simulink model "TypesOfSolverr"  (R2013a)
settings: Solver=FixedStepDiscrete  StartTime=0  StopTime=20  FixedStep=1  MaxStep=1  RelTol=1e-3
settings Model: Creator=ajdin  LastModifiedBy=ajdin
settings DataIOCC: LoadExternalInput=on

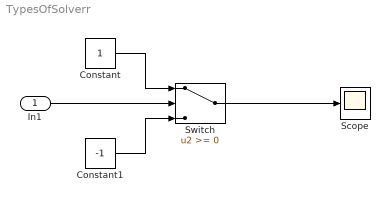
== system TypesOfSolverr ==
  In1 : Inport
  Constant : Constant
  Constant1 : Constant  Value=-1
  Scope : Scope
      settings: YMin=-3  YMax=3
  Switch : Switch
  wires:
  Switch/1 -> Scope/1
  In1/1 -> Switch/2
  Constant1/1 -> Switch/3
  Constant/1 -> Switch/1
